simulink model "L3Pilot_ADF_v1"  (R2018b)
settings: Solver=FixedStepAuto  StartTime=0.0  StopTime=350  RelTol=1e-3  EnableMultiTasking=on
values from neighbouring files (symbols this model uses):
  a_x_MRM_critical = 5    [Var_L3Pilot_ADF_v1.m]
  a_x_MRM_normal = 2    [Var_L3Pilot_ADF_v1.m]
  Distance_forced_lane_change = 10    [Var_L3Pilot_ADF_v1.m]
  K_d_value_100 = 0.09    [Var_L3Pilot_ADF_v1.m]
  K_d_value_130 = 0.08    [Var_L3Pilot_ADF_v1.m]
  K_d_value_60 = 0.1    [Var_L3Pilot_ADF_v1.m]
  K_i_value_100 = 1    [Var_L3Pilot_ADF_v1.m]
  K_i_value_130 = 1    [Var_L3Pilot_ADF_v1.m]
  K_i_value_60 = 1    [Var_L3Pilot_ADF_v1.m]
  K_p_value_100 = 0.1    [Var_L3Pilot_ADF_v1.m]
  K_p_value_130 = 0.1    [Var_L3Pilot_ADF_v1.m]
  K_p_value_60 = 0.1    [Var_L3Pilot_ADF_v1.m]
  K_v1_value_100 = 0.1    [Var_L3Pilot_ADF_v1.m]
  K_v1_value_130 = 0.1    [Var_L3Pilot_ADF_v1.m]
  K_v1_value_60 = 0.1    [Var_L3Pilot_ADF_v1.m]
  K_v2_value_100 = 0.2    [Var_L3Pilot_ADF_v1.m]
  K_v2_value_130 = 0.2    [Var_L3Pilot_ADF_v1.m]
  K_v2_value_60 = 0.2    [Var_L3Pilot_ADF_v1.m]
  Set_velocity = 60/3.6    (= 16.6666666667)    [Var_L3Pilot_ADF_v1.m]
  t_MRM = 60    [Var_L3Pilot_ADF_v1.m]
  t_takeover = 70    [Var_L3Pilot_ADF_v1.m]
  Tabt = 0.1    [Var_L3Pilot_ADF_v1.m]
  x_LC_Forced_value = 99999    [Var_L3Pilot_ADF_v1.m]
undefined symbols (not defined in the file or in its folder): ComponentState
libraries: simulink x2
(part 1 of 2)
settings Model: Creator=QXV8396  LastModifiedBy=Q395473
settings DataIOCC: LimitDataPoints=on
settings DebuggingCC: AllowSymbolicDim=off  SFUnexpectedBacktrackingDiag=warning  SFNoUnconditionalDefaultTransitionDiag=warning  SFExecutionAtInitializationDiag=none
settings ModelReferenceCC: PropagateSignalLabelsOutOfModel=off
settings SFSimCC: SimUseLocalCustomCode=off
settings RTWCC: SystemTargetFile=fmu_cs1.tlc  MakeCommand=make_rtw FMIT_INTERMEDIATE_LIB_DIR=DEFAULT FMIT_ADDITIONAL_CFLAGS=  TemplateMakefile=fmu_cs1_default_tmf  Description=FMU Co-Simulation 1.0 Standalone  RTWUseLocalCustomCode=off
settings CodeAppCC: StateflowObjectComments=on
settings STFCustomTargetCC: ModelReferenceCompliant=off  MultiInstanceERTCode=on  CodeInterfacePackaging=Reusable function  MATLABClassNameForMDSCustomization=Simulink.SoftwareTarget.TargetSpecificTriggerConfigurationBase  GRTInterface=on  GenerateAllocFcn=on  SystemTargetFile=fmu_cs1.tlc
settings ConfigComp: CovMetricSettings=dw  CovHtmlReporting=on  CovSaveCumulativeToWorkspaceVar=on  CovSaveSingleToWorkspaceVar=on  CovExternalEMLEnable=off

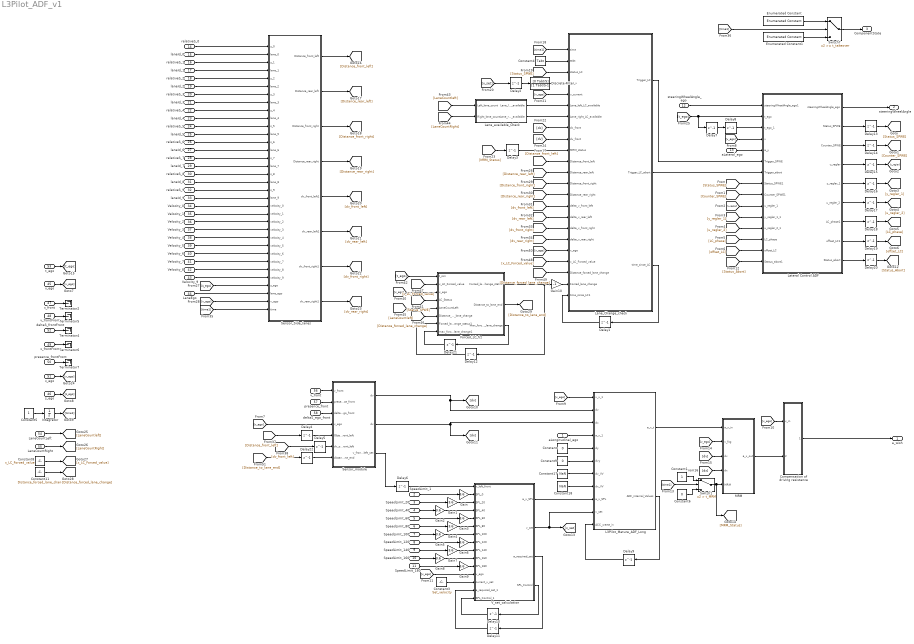
== system L3Pilot_ADF_v1 ==
  aLongitudinal_ego : Inport
  SpeedLimit_1 : Inport  Port=2  OutDataTypeStr=double
  SpeedLimit_20 : Inport  Port=3  OutDataTypeStr=double
  SpeedLimit_40 : Inport  Port=4  OutDataTypeStr=double
  SpeedLimit_60 : Inport  Port=5  OutDataTypeStr=double
  SpeedLimit_80 : Inport  Port=6  OutDataTypeStr=double
  SpeedLimit_100 : Inport  Port=7  OutDataTypeStr=double
  SpeedLimit_120 : Inport  Port=8  OutDataTypeStr=double
  SpeedLimit_140 : Inport  Port=9  OutDataTypeStr=double
  SpeedLimit_160 : Inport  Port=10  OutDataTypeStr=double
  SpeedLimit_180 : Inport  Port=11  OutDataTypeStr=double
  steeringWheelAngle_ego : Inport  Port=12
  aLateral_ego : Inport  Port=13
  relativeS_0 : Inport  Port=14  OutDataTypeStr=double
  laneId_0 : Inport  Port=15  OutDataTypeStr=int8
  relativeS_1 : Inport  Port=16  OutDataTypeStr=double
  laneId_1 : Inport  Port=17  OutDataTypeStr=int8
  relativeS_2 : Inport  Port=18  OutDataTypeStr=double
  laneId_2 : Inport  Port=19  OutDataTypeStr=int8
  relativeS_3 : Inport  Port=20  OutDataTypeStr=double
  laneId_3 : Inport  Port=21  OutDataTypeStr=int8
  relativeS_4 : Inport  Port=22  OutDataTypeStr=double
  laneId_4 : Inport  Port=23  OutDataTypeStr=int8
  relativeS_5 : Inport  Port=24  OutDataTypeStr=double
  laneId_5 : Inport  Port=25  OutDataTypeStr=int8
  relativeS_6 : Inport  Port=26  OutDataTypeStr=double
  laneId_6 : Inport  Port=27  OutDataTypeStr=int8
  relativeS_7 : Inport  Port=28  OutDataTypeStr=double
  laneId_7 : Inport  Port=29  OutDataTypeStr=int8
  relativeS_8 : Inport  Port=30  OutDataTypeStr=double
  laneId_8 : Inport  Port=31  OutDataTypeStr=int8
  relativeS_9 : Inport  Port=32  OutDataTypeStr=double
  laneId_9 : Inport  Port=33  OutDataTypeStr=int8
  Velocity_0 : Inport  Port=34  OutDataTypeStr=double
  Velocity_1 : Inport  Port=35  OutDataTypeStr=double
  Velocity_2 : Inport  Port=36  OutDataTypeStr=double
  Velocity_3 : Inport  Port=37  OutDataTypeStr=double
  Velocity_4 : Inport  Port=38  OutDataTypeStr=double
  Velocity_5 : Inport  Port=39  OutDataTypeStr=double
  Velocity_6 : Inport  Port=40  OutDataTypeStr=double
  Velocity_7 : Inport  Port=41  OutDataTypeStr=double
  Velocity_8 : Inport  Port=42  OutDataTypeStr=double
  Velocity_9 : Inport  Port=43  OutDataTypeStr=double
  LaneEgo : Inport  Port=44  OutDataTypeStr=int8
  v_ego : Inport  Port=45  OutDataTypeStr=double
  s_ego : Inport  Port=46
  x_front : Inport  Port=47  OutDataTypeStr=double
  v_frontFront : Inport  Port=48  OutDataTypeStr=double
  x_frontFront : Inport  Port=49  OutDataTypeStr=double
  presence_frontFront : Inport  Port=50  OutDataTypeStr=boolean
  x_ego : Inport  Port=51
  deltaS_frontFront : Inport  Port=52  OutDataTypeStr=double
  t_ego : Inport  Port=53
  LaneCountLeft : Inport  Port=54  OutDataTypeStr=int8
  LaneCountRight : Inport  Port=55  OutDataTypeStr=int8
  v_front : Inport  Port=56  OutDataTypeStr=double
  presence_front : Inport  Port=57  OutDataTypeStr=boolean
  deltaS_ego_front : Inport  Port=58
  Compensation of driving resistance : Subsystem
  Constant : Constant  Value=0  SampleTime=Tabt
  Constant1 : Constant  SampleTime=Tabt
  Constant11 : Constant  Value=Distance_forced_lane_change  SampleTime=Tabt
  Constant17 : Constant  Value=NaN  SampleTime=Tabt
  Constant18 : Constant  Value=NaN  SampleTime=Tabt
  Constant3 : Constant  Value=Set_velocity  SampleTime=Tabt
  Constant4 : Constant  Value=Tabt
  Constant5 : Constant  SampleTime=Tabt
  Constant6 : Constant  Value=0  SampleTime=Tabt
  Constant8 : Constant  Value=x_LC_Forced_value  SampleTime=Tabt
  Constant9 : Constant  Value=0  SampleTime=Tabt
  Delay{1..8,12..22} (19 alike) : Delay  DelayLength=1  InitialCondition=0  SampleTime=0.1
  Delay10 : Delay  DelayLength=1  InitialCondition=0  SampleTime=Tabt
  Delay11 : Delay  DelayLength=1  InitialCondition=0  SampleTime=Tabt
  Delay9 : Delay  DelayLength=1  InitialCondition=0  SampleTime=Tabt
  Discrete Filter : DiscreteFilter  Numerator=[0 Tabt/5]  Denominator=[1 Tabt/5-1]
  Enumerated Constant : simulink/Sources/Enumerated Constant  OutDataTypeStr=Enum: ComponentState  Value=ComponentState.Disabled  SampleTime=inf
      settings: SourceProductName=Simulink
  Enumerated Constant1 : simulink/Sources/Enumerated Constant  OutDataTypeStr=Enum: ComponentState  Value=ComponentState.Acting  SampleTime=inf
      settings: SourceProductName=Simulink
  Forced_LC_fct : MATLAB Function  TreatAsAtomicUnit=on
  Gain{,1..9} (10 alike) : Gain  Gain=3.6
  Gain10 : Gain  Gain=-1
  Integrator : Integrator
  L3Pilot_Mature_ADF_Long : Subsystem
  Lane_Change_check : MATLAB Function  TreatAsAtomicUnit=on
  Lane_available_Check : Subsystem
  Lateral Control ADF : MATLAB Function  TreatAsAtomicUnit=on
  MRM : Subsystem
  Sensor_Side_lanes : Subsystem
  Sensor_module : Subsystem
  Switch1 : Switch  Criteria=u2 > Threshold  Threshold=t_MRM
  Switch7 : Switch  Threshold=t_takeover
  Terminator{2,4..7} (5 alike) : Terminator
  V_set_calculation : MATLAB Function  TreatAsAtomicUnit=on
  a_wish : Outport
  steeringWheelAngle : Outport  Port=2
  ComponentState : Outport  Port=3  OutDataTypeStr=Enum: ComponentState
  wires:
  Constant17/1 -> L3Pilot_Mature_ADF_Long/7(dv_VV)
  Constant18/1 -> L3Pilot_Mature_ADF_Long/8(dx_VV)
  Constant9/1 -> L3Pilot_Mature_ADF_Long/6(dvy)
  L3Pilot_Mature_ADF_Long/1(a_x_t) -> MRM/1(a_x_in)
  Constant/1 -> L3Pilot_Mature_ADF_Long/5(dy)
  Delay9/1 -> L3Pilot_Mature_ADF_Long/11(ACC_werte_in)
  aLongitudinal_ego/1 -> L3Pilot_Mature_ADF_Long/4("a_x_1 ")
  L3Pilot_Mature_ADF_Long/2(ADF_internal_Values) -> Delay9/1
  [v_ego] -> L3Pilot_Mature_ADF_Long/1(v_x_1)
  [v_ego] -> Compensation of driving resistance/1(v_in)
  Sensor_module/1(dv) -> L3Pilot_Mature_ADF_Long/2(dv), [dv]
  Sensor_module/2(dx) -> L3Pilot_Mature_ADF_Long/3(dx), [dx]
  V_set_calculation/2(v_set) -> L3Pilot_Mature_ADF_Long/10(v_set), [v_set]
  Delay10/1 -> V_set_calculation/15(SPL_Control_1)
  Constant1/1 -> Switch1/1
  [time1] -> Switch1/2
  Constant6/1 -> Switch1/3
  Switch1/1 -> [MRM_Status], MRM/5(MRM)
  MRM/1(a_x_out) -> Compensation of driving resistance/2(a_x_in)
  [v_ego] -> MRM/2(v_fzg)
  [dx] -> MRM/4(dx)
  [dv] -> MRM/3(dv)
  V_set_calculation/4(SPL_Control) -> Delay10/1
  V_set_calculation/3(a_required_set) -> Delay11/1
  Delay11/1 -> V_set_calculation/14(a_required_set_1)
  [v_ego] -> V_set_calculation/12(v_ego)
  SpeedLimit_1/1 -> Gain/1
  SpeedLimit_20/1 -> Gain1/1
  SpeedLimit_40/1 -> Gain2/1
  SpeedLimit_60/1 -> Gain3/1
  SpeedLimit_80/1 -> Gain4/1
  SpeedLimit_100/1 -> Gain5/1
  SpeedLimit_120/1 -> Gain6/1
  SpeedLimit_160/1 -> Gain8/1
  SpeedLimit_180/1 -> Gain9/1
  SpeedLimit_140/1 -> Gain7/1
  Constant3/1 -> V_set_calculation/13(current_v_set)
  V_set_calculation/1(a_x_SPL) -> L3Pilot_Mature_ADF_Long/9(a_x_SPL)
  Gain/1 -> V_set_calculation/2(SPL_0)
  Gain1/1 -> V_set_calculation/3(SPL_20)
  Gain2/1 -> V_set_calculation/4(SPL_40)
  Gain3/1 -> V_set_calculation/5(SPL_60)
  Gain4/1 -> V_set_calculation/6(SPL_80)
  Gain5/1 -> V_set_calculation/7(SPL_100)
  Gain6/1 -> V_set_calculation/8(SPL_120)
  Gain7/1 -> V_set_calculation/9(SPL_140)
  Gain8/1 -> V_set_calculation/10(SPL_160)
  Gain9/1 -> V_set_calculation/11(SPL_180)
  Sensor_module/3(v_front_left_set) -> Delay6/1
  Delay6/1 -> V_set_calculation/1(v_left_front)
  Compensation of driving resistance/1(a_x_out) -> a_wish/1
  [t_ego] -> Forced_LC_fct/1(t_sim)
  [LaneCountleft] -> Lane_available_Check/1(Left_lane_count)
  Gain10/1 -> Lane_Change_check/22(Forced_lane_change)
  relativeS_1/1 -> Sensor_Side_lanes/3(s_1)
  Delay21/1 -> Forced_LC_fct/8(max_force_lane_change1)
  Velocity_2/1 -> Sensor_Side_lanes/23(velocity_2)
  laneId_9/1 -> Sensor_Side_lanes/20(lane_9)
  Forced_LC_fct/3(max_force_lane_change) -> Delay21/1
  relativeS_4/1 -> Sensor_Side_lanes/9(s_4)
  [dv] -> Lane_Change_check/9(dv_front)
  [Status_SPWE] -> Forced_LC_fct/4(LC_Status)
  Forced_LC_fct/1(Forced_lane_change_status) -> Delay12/1, Gain10/1
  Lateral Control ADF/4(u_regler) -> Delay15/1
  Delay12/1 -> Forced_LC_fct/7(Forced_lane_change_status1)
  [time1] -> Switch7/2
  Constant4/1 -> Lane_Change_check/2(tabt)
  [Distance_rear_left] -> Lane_Change_check/12(Distance_rear_left)
  Velocity_4/1 -> Sensor_Side_lanes/25(velocity_4)
  [Distance_rear_right] -> Lane_Change_check/14(Distance_rear_right)
  [dv_front_right] -> Lane_Change_check/17(delta_v_front_right)
  Sensor_Side_lanes/4(Distance_rear_right) -> [Distance_rear_right]
  Sensor_Side_lanes/2(Distance_rear_left) -> [Distance_rear_left]
  [time1] -> Lane_Change_check/1(time)
  Switch7/1 -> ComponentState/1
  [Status_Abort] -> Lateral Control ADF/15(Status_abort1)
  Lateral Control ADF/3(Counter_SPWE) -> Delay14/1
  Sensor_Side_lanes/6(dv_rear_left1) -> [dv_rear_left]
  Velocity_8/1 -> Sensor_Side_lanes/29(velocity_8)
  Velocity_9/1 -> Sensor_Side_lanes/30(velocity_9)
  [Distance_front_left] -> Lane_Change_check/11(Distance_front_left)
  relativeS_8/1 -> Sensor_Side_lanes/17(s_8)
  Sensor_Side_lanes/5(dv_front_left1) -> [dv_front_left]
  [Distance_front_right] -> Lane_Change_check/13(Distance_front_right)
  [v_set] -> Delay2/1
  Sensor_Side_lanes/3(Distance_front_right) -> [Distance_front_right]
  relativeS_2/1 -> Sensor_Side_lanes/5(s_2)
  relativeS_9/1 -> Sensor_Side_lanes/19(s_9)
  Velocity_1/1 -> Sensor_Side_lanes/22(velocity_1)
  Delay19/1 -> [offset_LC]
  relativeS_7/1 -> Sensor_Side_lanes/15(s_7)
  relativeS_6/1 -> Sensor_Side_lanes/13(s_6)
  relativeS_0/1 -> Sensor_Side_lanes/1(s_0)
  laneId_7/1 -> Sensor_Side_lanes/16(lane_7)
  relativeS_5/1 -> Sensor_Side_lanes/11(s_5)
  laneId_2/1 -> Sensor_Side_lanes/6(lane_2)
  laneId_3/1 -> Sensor_Side_lanes/8(lane_3)
  laneId_1/1 -> Sensor_Side_lanes/4(lane_1)
  Delay1/1 -> Lane_Change_check/23(time_since_LC1)
  Lateral Control ADF/8(offset_LC1) -> Delay19/1
  Delay3/1 -> Lane_Change_check/10(MRM_status)
  Delay14/1 -> [Counter_SPWE]
  Delay7/1 -> Delay8/1
  Delay15/1 -> [u_regler]
  Lateral Control ADF/7(LC_phase1) -> Delay18/1
  Delay20/1 -> [Status_Abort]
  Delay2/1 -> Discrete Filter/1
  [Status_SPWE] -> Lane_Change_check/3(status_LC)
  Delay16/1 -> [y_regler_1]
  [MRM_Status] -> Delay3/1
  Velocity_3/1 -> Sensor_Side_lanes/24(velocity_3)
  Lateral Control ADF/2(Status_SPWE) -> Delay13/1
  Velocity_6/1 -> Sensor_Side_lanes/27(velocity_6)
  Delay13/1 -> [Status_SPWE]
  aLateral_ego/1 -> Lateral Control ADF/5(a_y)
  [v_ego] -> Sensor_Side_lanes/33(v_ego)
  Lane_Change_check/1(Trigger_LC) -> Lateral Control ADF/6(Trigger_SPWE)
  Lateral Control ADF/6(u_regler_2) -> Delay17/1
  [u_regler_2] -> Lateral Control ADF/12(u_regler_2_1)
  LaneEgo/1 -> Sensor_Side_lanes/32(lane_ego)
  [v_ego] -> Lane_Change_check/5(v_current)
  Lateral Control ADF/5(y_regler_1) -> Delay16/1
  Velocity_7/1 -> Sensor_Side_lanes/28(velocity_7)
  [x_ego] -> Forced_LC_fct/3(x_ego)
  [y_regler_1] -> Lateral Control ADF/11(y_regler_1_1)
  [x_LC_Forced_value] -> Lane_Change_check/20(x_LC_Forced_value)
  Delay8/1 -> Lateral Control ADF/3(t_ego_1)
  [v_ego] -> Lateral Control ADF/4(v)
  Delay18/1 -> [LC_phase]
  [dv_rear_right] -> Lane_Change_check/18(delta_v_rear_right)
  Velocity_5/1 -> Sensor_Side_lanes/26(velocity_5)
  [Status_SPWE] -> Lateral Control ADF/8(Status_SPWE1)
  Lane_available_Check/1(Lane_left_LC_available) -> Lane_Change_check/6(Lane_left_LC_available)
  relativeS_3/1 -> Sensor_Side_lanes/7(s_3)
  Sensor_Side_lanes/1(Distance_front_left) -> [Distance_front_left]
  laneId_6/1 -> Sensor_Side_lanes/14(lane_6)
  [x_LC_Forced_value] -> Forced_LC_fct/2(x_LC_Forced_value)
  [offset_LC] -> Lateral Control ADF/14(offset_LC)
  Delay17/1 -> [u_regler_2]
  [t_ego] -> Delay7/1, Lateral Control ADF/2(t_ego)
  Lane_available_Check/2(Lane_right_LC_available) -> Lane_Change_check/7(Lane_right_LC_available)
  [LaneCountRight] -> Lane_available_Check/2(Right_lane_count)
  Lane_Change_check/3(time_since_LC) -> Delay1/1
  [x_ego] -> Lane_Change_check/19(x_ego)
  Lateral Control ADF/9(Status_abort) -> Delay20/1
  [dv_front_left] -> Lane_Change_check/15(delta_v_front_left)
  Sensor_Side_lanes/8(dv_rear_right1) -> [dv_rear_right]
  Lateral Control ADF/1(steeringWheelAngle_ego) -> steeringWheelAngle/1
  Lane_Change_check/2(Trigger_LC_abort) -> Lateral Control ADF/7(Trigger_abort)
  laneId_8/1 -> Sensor_Side_lanes/18(lane_8)
  [time1] -> Sensor_Side_lanes/34(time)
  [LC_phase] -> Lateral Control ADF/13(LC_phase)
  Discrete Filter/1 -> Lane_Change_check/4(set_v)
  [u_regler] -> Lateral Control ADF/10(u_regler_1)
  [dx] -> Lane_Change_check/8(dx_front)
  [dv_rear_left] -> Lane_Change_check/16(delta_v_rear_left)
  [Distance_forced_lane_change] -> Forced_LC_fct/6(Distance_forced_lane_change)
  steeringWheelAngle_ego/1 -> Lateral Control ADF/1(steeringWheelAngle_ego1)
  [s_ego] -> Sensor_Side_lanes/31("s_ego ")
  Sensor_Side_lanes/7(dv_front_right1) -> [dv_front_right]
  laneId_4/1 -> Sensor_Side_lanes/10(lane_4)
  Enumerated Constant1/1 -> Switch7/3
  Enumerated Constant/1 -> Switch7/1
  Forced_LC_fct/2(Distance_to_lane_end) -> [Distance_to_lane_end]
  laneId_5/1 -> Sensor_Side_lanes/12(lane_5)
  [Counter_SPWE] -> Lateral Control ADF/9(Counter_SPWE1)
  [LaneCountleft] -> Forced_LC_fct/5(LaneCountLeft)
  [Distance_forced_lane_change] -> Lane_Change_check/21(Distance_forced_lane_change)
  laneId_0/1 -> Sensor_Side_lanes/2("lane_0 ")
  Velocity_0/1 -> Sensor_Side_lanes/21(velocity_0)
  x_front/1 -> Terminator2/1
  t_ego/1 -> [t_ego]
  x_frontFront/1 -> Terminator6/1
  x_ego/1 -> [x_ego]
  Integrator/1 -> [time1]
  s_ego/1 -> [s_ego]
  Constant5/1 -> Integrator/1
  deltaS_frontFront/1 -> Terminator4/1
  LaneCountLeft/1 -> [LaneCountleft]
  LaneCountRight/1 -> [LaneCountRight]
  v_frontFront/1 -> Terminator5/1
  Constant8/1 -> [x_LC_Forced_value]
  v_ego/1 -> [v_ego]
  Constant11/1 -> [Distance_forced_lane_change]
  presence_frontFront/1 -> Terminator7/1
  Delay4/1 -> Sensor_module/5("Object_front_left ")
  Delay5/1 -> Sensor_module/6(dv_object_front_left)
  v_front/1 -> Sensor_module/1(v_front)
  [v_ego] -> Sensor_module/4(v_ego)
  presence_front/1 -> Sensor_module/2(presence_front)
  [Distance_to_lane_end] -> Delay22/1
  [dv_front_left] -> Delay5/1
  Delay22/1 -> Sensor_module/7(distance_lane_end)
  deltaS_ego_front/1 -> Sensor_module/3(deltaS_ego_front)
  [Distance_front_left] -> Delay4/1

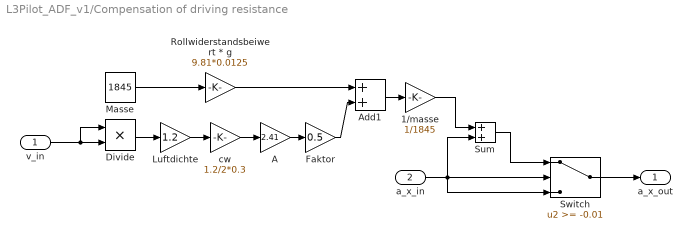
== system L3Pilot_ADF_v1/Compensation of driving resistance ==
  v_in : Inport
  a_x_in : Inport  Port=2
  1/masse : Gain  Gain=1/1845
  A : Gain  Gain=2.41  OutDataTypeStr=double
  Add1 : Sum
  Divide : Product  Inputs=**
  Faktor : Gain  Gain=0.5  OutDataTypeStr=double
  Luftdichte : Gain  Gain=1.2  OutDataTypeStr=double
  Masse : Constant  Value=1845
  Rollwiderstandsbeiwert * g : Gain  Gain=9.81*0.0125
  Sum : Sum
  Switch : Switch  Threshold=-0.01
  cw : Gain  Gain=1.2/2*0.3  OutDataTypeStr=double
  a_x_out : Outport
  wires:
  Divide/1 -> Luftdichte/1
  Add1/1 -> 1/masse/1
  a_x_in/1 -> Sum/2, Switch/3, Switch/2
  Switch/1 -> a_x_out/1
  Masse/1 -> Rollwiderstandsbeiwert * g/1
  v_in/1 -> Divide/1, Divide/2
  1/masse/1 -> Sum/1
  Sum/1 -> Switch/1
  Rollwiderstandsbeiwert * g/1 -> Add1/1
  cw/1 -> A/1
  Luftdichte/1 -> cw/1
  A/1 -> Faktor/1
  Faktor/1 -> Add1/2

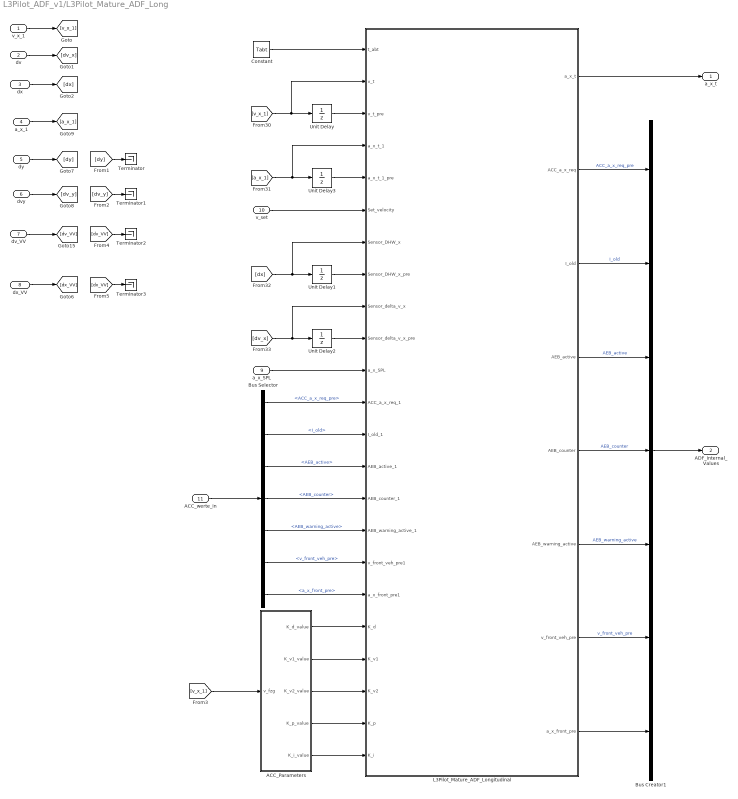
== system L3Pilot_ADF_v1/L3Pilot_Mature_ADF_Long ==
  v_x_1 : Inport
  dv : Inport  Port=2
  dx : Inport  Port=3
  "a_x_1 " : Inport  Port=4
  dy : Inport  Port=5
  dvy : Inport  Port=6
  dv_VV : Inport  Port=7
  dx_VV : Inport  Port=8
  a_x_SPL : Inport  Port=9
  v_set : Inport  Port=10
  ACC_werte_in : Inport  Port=11
  ACC_Parameters : Subsystem
  Bus Creator1 : BusCreator  Inputs=7
  Bus Selector : BusSelector  OutputSignals=ACC_a_x_req_pre,I_old,AEB_active,AEB_counter,AEB_warning_active,v_front_veh_pre,a_x_front_pre
  Constant : Constant  Value=Tabt
  L3Pilot_Mature_ADF_Longitudinal : MATLAB Function  TreatAsAtomicUnit=on
  Terminator{,1..3} (4 alike) : Terminator
  Unit Delay{,1..3} (4 alike) : UnitDelay  SampleTime=-1
  a_x_t : Outport
  ADF_internal_Values : Outport  Port=2
  wires:
  v_x_1/1 -> [v_x_1]
  dv/1 -> [dv_x]
  dx/1 -> [dx]
  dy/1 -> [dy]
  dvy/1 -> [dv_y]
  "a_x_1 "/1 -> [a_x_1]
  Bus Creator1/1 -> ADF_internal_Values/1
  ACC_werte_in/1 -> Bus Selector/1
  Constant/1 -> L3Pilot_Mature_ADF_Longitudinal/1(t_abt)
  [v_x_1] -> L3Pilot_Mature_ADF_Longitudinal/2(v_t), Unit Delay/1
  Unit Delay/1 -> L3Pilot_Mature_ADF_Longitudinal/3(v_t_pre)
  [a_x_1] -> L3Pilot_Mature_ADF_Longitudinal/4(a_x_t_1), Unit Delay3/1
  v_set/1 -> L3Pilot_Mature_ADF_Longitudinal/6(Set_velocity)
  L3Pilot_Mature_ADF_Longitudinal/1(a_x_t) -> a_x_t/1
  [dx] -> L3Pilot_Mature_ADF_Longitudinal/7(Sensor_DHW_x), Unit Delay1/1
  [dv_x] -> L3Pilot_Mature_ADF_Longitudinal/9(Sensor_delta_v_x), Unit Delay2/1
  Unit Delay1/1 -> L3Pilot_Mature_ADF_Longitudinal/8(Sensor_DHW_x_pre)
  Unit Delay2/1 -> L3Pilot_Mature_ADF_Longitudinal/10(Sensor_delta_v_x_pre)
  dx_VV/1 -> [dx_VV]
  dv_VV/1 -> [dv_VV]
  L3Pilot_Mature_ADF_Longitudinal/2(ACC_a_x_req) -> Bus Creator1/1  "ACC_a_x_req_pre"
  Bus Selector/2 -> L3Pilot_Mature_ADF_Longitudinal/13(I_old_1)  "<I_old>"
  [dy] -> Terminator/1
  [dv_y] -> Terminator1/1
  L3Pilot_Mature_ADF_Longitudinal/3(I_old) -> Bus Creator1/2  "I_old"
  Bus Selector/1 -> L3Pilot_Mature_ADF_Longitudinal/12(ACC_a_x_req_1)  "<ACC_a_x_req_pre>"
  ACC_Parameters/1(K_d_value) -> L3Pilot_Mature_ADF_Longitudinal/19(K_d)
  ACC_Parameters/2(K_v1_value) -> L3Pilot_Mature_ADF_Longitudinal/20(K_v1)
  ACC_Parameters/3(K_v2_value) -> L3Pilot_Mature_ADF_Longitudinal/21(K_v2)
  ACC_Parameters/4(K_p_value) -> L3Pilot_Mature_ADF_Longitudinal/22(K_p)
  ACC_Parameters/5(K_i_value) -> L3Pilot_Mature_ADF_Longitudinal/23(K_i)
  L3Pilot_Mature_ADF_Longitudinal/4(AEB_active) -> Bus Creator1/3  "AEB_active"
  L3Pilot_Mature_ADF_Longitudinal/5(AEB_counter) -> Bus Creator1/4  "AEB_counter"
  Bus Selector/3 -> L3Pilot_Mature_ADF_Longitudinal/14(AEB_active_1)  "<AEB_active>"
  Bus Selector/4 -> L3Pilot_Mature_ADF_Longitudinal/15(AEB_counter_1)  "<AEB_counter>"
  Unit Delay3/1 -> L3Pilot_Mature_ADF_Longitudinal/5(a_x_t_1_pre)
  L3Pilot_Mature_ADF_Longitudinal/6(AEB_warning_active) -> Bus Creator1/5  "AEB_warning_active"
  Bus Selector/5 -> L3Pilot_Mature_ADF_Longitudinal/16(AEB_warning_active_1)  "<AEB_warning_active>"
  [v_x_1] -> ACC_Parameters/1(v_fzg)
  [dv_VV] -> Terminator2/1
  [dx_VV] -> Terminator3/1
  L3Pilot_Mature_ADF_Longitudinal/7(v_front_veh_pre) -> Bus Creator1/6  "v_front_veh_pre"
  Bus Selector/6 -> L3Pilot_Mature_ADF_Longitudinal/17(v_front_veh_pre1)  "<v_front_veh_pre>"
  L3Pilot_Mature_ADF_Longitudinal/8(a_x_front_pre) -> Bus Creator1/7
  Bus Selector/7 -> L3Pilot_Mature_ADF_Longitudinal/18(a_x_front_pre1)  "<a_x_front_pre>"
  a_x_SPL/1 -> L3Pilot_Mature_ADF_Longitudinal/11(a_x_SPL)

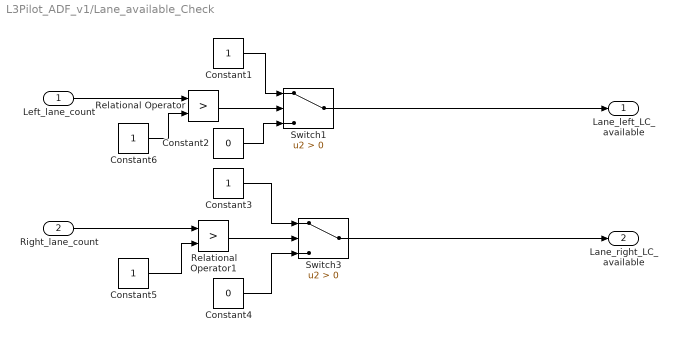
== system L3Pilot_ADF_v1/Lane_available_Check ==
  Left_lane_count : Inport
  Right_lane_count : Inport  Port=2
  Constant{1,3,5..6} (4 alike) : Constant  SampleTime=Tabt
  Constant2 : Constant  Value=0  SampleTime=Tabt
  Constant4 : Constant  Value=0  SampleTime=Tabt
  Relational Operator : RelationalOperator  Operator=>  OutDataTypeStr=boolean  RndMeth=Simplest
  Relational Operator1 : RelationalOperator  Operator=>  OutDataTypeStr=boolean  RndMeth=Simplest
  Switch1 : Switch  Criteria=u2 > Threshold
  Switch3 : Switch  Criteria=u2 > Threshold
  Lane_left_LC_available : Outport
  Lane_right_LC_available : Outport  Port=2
  wires:
  Constant2/1 -> Switch1/3
  Constant1/1 -> Switch1/1
  Constant3/1 -> Switch3/1
  Constant4/1 -> Switch3/3
  Constant6/1 -> Relational Operator/2
  Relational Operator/1 -> Switch1/2
  Relational Operator1/1 -> Switch3/2
  Constant5/1 -> Relational Operator1/2
  Right_lane_count/1 -> Relational Operator1/1
  Left_lane_count/1 -> Relational Operator/1
  Switch1/1 -> Lane_left_LC_available/1
  Switch3/1 -> Lane_right_LC_available/1

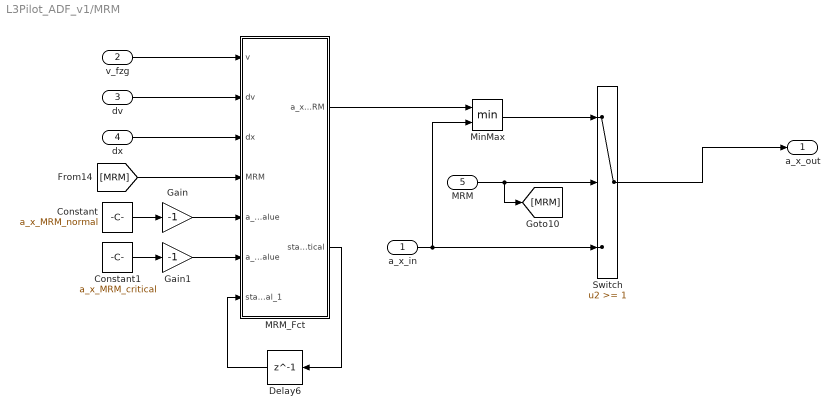
== system L3Pilot_ADF_v1/MRM ==
  a_x_in : Inport
  v_fzg : Inport  Port=2
  dv : Inport  Port=3
  dx : Inport  Port=4
  MRM : Inport  Port=5
  Constant : Constant  Value=a_x_MRM_normal  SampleTime=Tabt
  Constant1 : Constant  Value=a_x_MRM_critical  SampleTime=Tabt
  Delay6 : Delay  DelayLength=1  InitialCondition=0  SampleTime=0.1
  Gain : Gain  Gain=-1
  Gain1 : Gain  Gain=-1
  MRM_Fct : MATLAB Function  TreatAsAtomicUnit=on
  MinMax : MinMax  Inputs=2
  Switch : Switch  Threshold=1
  a_x_out : Outport
  wires:
  MRM/1 -> [MRM], Switch/2
  Switch/1 -> a_x_out/1
  a_x_in/1 -> MinMax/2, Switch/3
  MinMax/1 -> Switch/1
  MRM_Fct/1(a_x_MRM) -> MinMax/1
  v_fzg/1 -> MRM_Fct/1(v)
  dv/1 -> MRM_Fct/2(dv)
  dx/1 -> MRM_Fct/3(dx)
  [MRM] -> MRM_Fct/4(MRM)
  MRM_Fct/2(status_critical) -> Delay6/1
  Delay6/1 -> MRM_Fct/7(status_critical_1)
  Constant/1 -> Gain/1
  Constant1/1 -> Gain1/1
  Gain/1 -> MRM_Fct/5(a_x_MRM_normal_value)
  Gain1/1 -> MRM_Fct/6(a_x_MRM_critical_value)

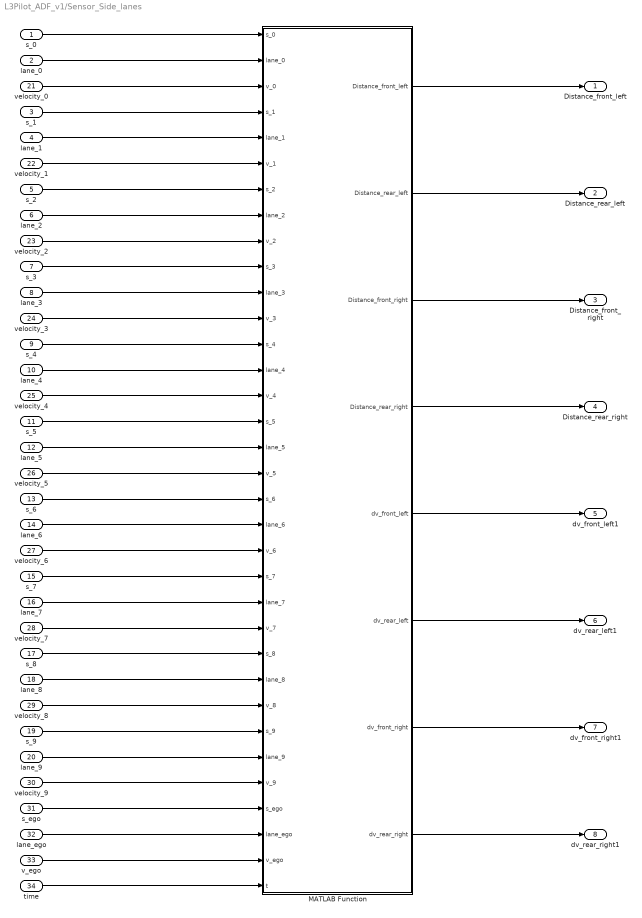
== system L3Pilot_ADF_v1/Sensor_Side_lanes ==
  s_0 : Inport
  "lane_0 " : Inport  Port=2
  s_1 : Inport  Port=3
  lane_1 : Inport  Port=4
  s_2 : Inport  Port=5
  lane_2 : Inport  Port=6
  s_3 : Inport  Port=7
  lane_3 : Inport  Port=8
  s_4 : Inport  Port=9
  lane_4 : Inport  Port=10
  s_5 : Inport  Port=11
  lane_5 : Inport  Port=12
  s_6 : Inport  Port=13
  lane_6 : Inport  Port=14
  s_7 : Inport  Port=15
  lane_7 : Inport  Port=16
  s_8 : Inport  Port=17
  lane_8 : Inport  Port=18
  s_9 : Inport  Port=19
  lane_9 : Inport  Port=20
  velocity_0 : Inport  Port=21
  velocity_1 : Inport  Port=22
  velocity_2 : Inport  Port=23
  velocity_3 : Inport  Port=24
  velocity_4 : Inport  Port=25
  velocity_5 : Inport  Port=26
  velocity_6 : Inport  Port=27
  velocity_7 : Inport  Port=28
  velocity_8 : Inport  Port=29
  velocity_9 : Inport  Port=30
  "s_ego " : Inport  Port=31
  lane_ego : Inport  Port=32
  v_ego : Inport  Port=33
  time : Inport  Port=34
  MATLAB Function : MATLAB Function  TreatAsAtomicUnit=on
  Distance_front_left : Outport
  Distance_rear_left : Outport  Port=2
  Distance_front_right : Outport  Port=3
  Distance_rear_right : Outport  Port=4
  dv_front_left1 : Outport  Port=5
  dv_rear_left1 : Outport  Port=6
  dv_front_right1 : Outport  Port=7
  dv_rear_right1 : Outport  Port=8
  wires:
  MATLAB Function/1(Distance_front_left) -> Distance_front_left/1
  MATLAB Function/2(Distance_rear_left) -> Distance_rear_left/1
  MATLAB Function/3(Distance_front_right) -> Distance_front_right/1
  MATLAB Function/4(Distance_rear_right) -> Distance_rear_right/1
  MATLAB Function/5(dv_front_left) -> dv_front_left1/1
  MATLAB Function/6(dv_rear_left) -> dv_rear_left1/1
  MATLAB Function/7(dv_front_right) -> dv_front_right1/1
  MATLAB Function/8(dv_rear_right) -> dv_rear_right1/1
  s_0/1 -> MATLAB Function/1(s_0)
  "lane_0 "/1 -> MATLAB Function/2(lane_0)
  s_1/1 -> MATLAB Function/4(s_1)
  lane_1/1 -> MATLAB Function/5(lane_1)
  s_2/1 -> MATLAB Function/7(s_2)
  lane_2/1 -> MATLAB Function/8(lane_2)
  s_3/1 -> MATLAB Function/10(s_3)
  lane_3/1 -> MATLAB Function/11(lane_3)
  s_4/1 -> MATLAB Function/13(s_4)
  lane_4/1 -> MATLAB Function/14(lane_4)
  s_5/1 -> MATLAB Function/16(s_5)
  lane_5/1 -> MATLAB Function/17(lane_5)
  s_6/1 -> MATLAB Function/19(s_6)
  lane_6/1 -> MATLAB Function/20(lane_6)
  s_7/1 -> MATLAB Function/22(s_7)
  lane_7/1 -> MATLAB Function/23(lane_7)
  s_8/1 -> MATLAB Function/25(s_8)
  lane_8/1 -> MATLAB Function/26(lane_8)
  s_9/1 -> MATLAB Function/28(s_9)
  lane_9/1 -> MATLAB Function/29(lane_9)
  "s_ego "/1 -> MATLAB Function/31(s_ego)
  lane_ego/1 -> MATLAB Function/32(lane_ego)
  velocity_0/1 -> MATLAB Function/3(v_0)
  velocity_1/1 -> MATLAB Function/6(v_1)
  velocity_2/1 -> MATLAB Function/9(v_2)
  velocity_3/1 -> MATLAB Function/12(v_3)
  velocity_4/1 -> MATLAB Function/15(v_4)
  velocity_5/1 -> MATLAB Function/18(v_5)
  velocity_6/1 -> MATLAB Function/21(v_6)
  velocity_7/1 -> MATLAB Function/24(v_7)
  velocity_8/1 -> MATLAB Function/27(v_8)
  velocity_9/1 -> MATLAB Function/30(v_9)
  v_ego/1 -> MATLAB Function/33(v_ego)
  time/1 -> MATLAB Function/34(t)

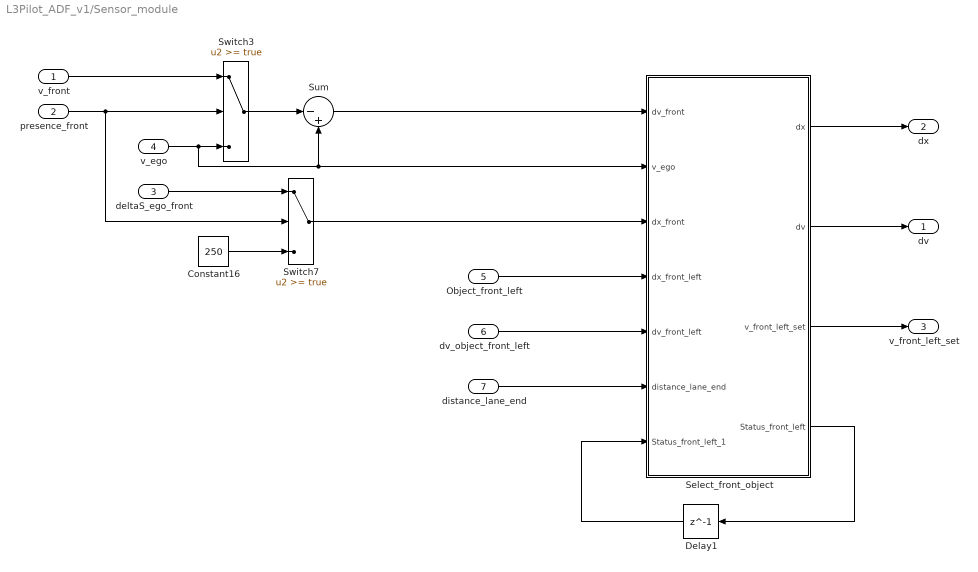
== system L3Pilot_ADF_v1/Sensor_module ==
  v_front : Inport
  presence_front : Inport  Port=2  OutDataTypeStr=boolean
  deltaS_ego_front : Inport  Port=3
  v_ego : Inport  Port=4  OutDataTypeStr=double
  "Object_front_left " : Inport  Port=5  OutDataTypeStr=double
  dv_object_front_left : Inport  Port=6  OutDataTypeStr=double
  distance_lane_end : Inport  Port=7  OutDataTypeStr=double
  Constant16 : Constant  Value=250  SampleTime=Tabt
  Delay1 : Delay  DelayLength=1  InitialCondition=0  SampleTime=0.1
  Select_front_object : MATLAB Function  TreatAsAtomicUnit=on
  Sum : Sum  Inputs=|-+
  Switch3 : Switch  Threshold=true
  Switch7 : Switch  Threshold=true
  dv : Outport
  dx : Outport  Port=2
  v_front_left_set : Outport  Port=3
  wires:
  v_front/1 -> Switch3/1
  Switch3/1 -> Sum/1
  Sum/1 -> Select_front_object/1(dv_front)
  deltaS_ego_front/1 -> Switch7/1
  presence_front/1 -> Switch7/2, Switch3/2
  Constant16/1 -> Switch7/3
  v_ego/1 -> Sum/2, Select_front_object/2(v_ego), Switch3/3
  Switch7/1 -> Select_front_object/3(dx_front)
  "Object_front_left "/1 -> Select_front_object/4(dx_front_left)
  dv_object_front_left/1 -> Select_front_object/5(dv_front_left)
  Select_front_object/1(dx) -> dx/1
  Select_front_object/2(dv) -> dv/1
  Select_front_object/3(v_front_left_set) -> v_front_left_set/1
  Select_front_object/4(Status_front_left) -> Delay1/1
  Delay1/1 -> Select_front_object/7(Status_front_left_1)
  distance_lane_end/1 -> Select_front_object/6(distance_lane_end)

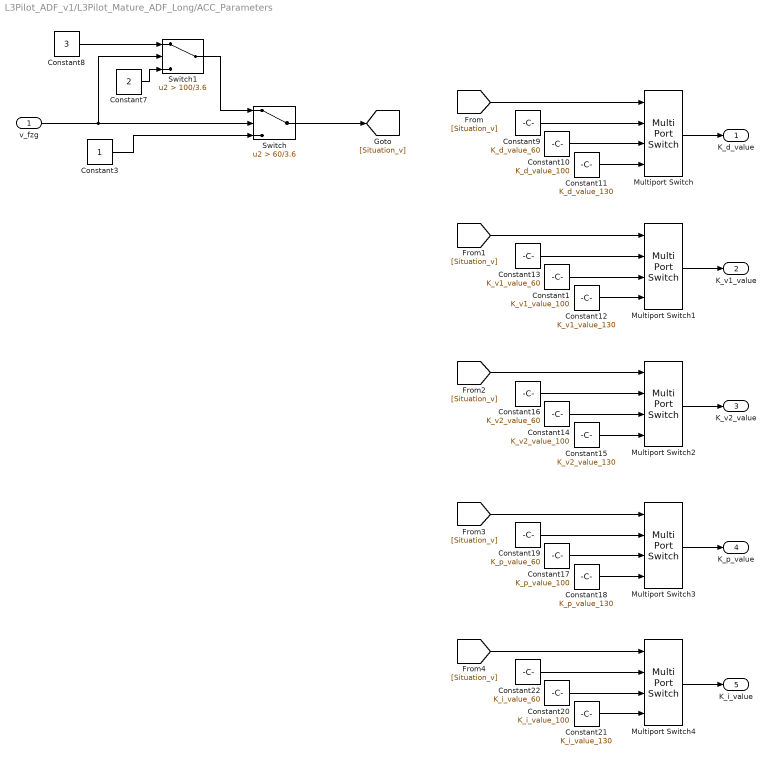
== system L3Pilot_ADF_v1/L3Pilot_Mature_ADF_Long/ACC_Parameters ==
  v_fzg : Inport
  Constant1 : Constant  Value=K_v1_value_100
  Constant10 : Constant  Value=K_d_value_100
  Constant11 : Constant  Value=K_d_value_130
  Constant12 : Constant  Value=K_v1_value_130
  Constant13 : Constant  Value=K_v1_value_60
  Constant14 : Constant  Value=K_v2_value_100
  Constant15 : Constant  Value=K_v2_value_130
  Constant16 : Constant  Value=K_v2_value_60
  Constant17 : Constant  Value=K_p_value_100
  Constant18 : Constant  Value=K_p_value_130
  Constant19 : Constant  Value=K_p_value_60
  Constant20 : Constant  Value=K_i_value_100
  Constant21 : Constant  Value=K_i_value_130
  Constant22 : Constant  Value=K_i_value_60
  Constant3 : Constant
  Constant7 : Constant  Value=2
  Constant8 : Constant  Value=3
  Constant9 : Constant  Value=K_d_value_60
  Multiport Switch{,1..4} (5 alike) : MultiPortSwitch
  Switch : Switch  Criteria=u2 > Threshold  Threshold=60/3.6
  Switch1 : Switch  Criteria=u2 > Threshold  Threshold=100/3.6
  K_d_value : Outport
  K_v1_value : Outport  Port=2
  K_v2_value : Outport  Port=3
  K_p_value : Outport  Port=4
  K_i_value : Outport  Port=5
  wires:
  v_fzg/1 -> Switch/2, Switch1/2
  Constant3/1 -> Switch/3
  Constant7/1 -> Switch1/3
  Constant8/1 -> Switch1/1
  Switch1/1 -> Switch/1
  Switch/1 -> [Situation_v]
  [Situation_v] -> Multiport Switch/1
  Constant9/1 -> Multiport Switch/2
  Constant10/1 -> Multiport Switch/3
  Constant11/1 -> Multiport Switch/4
  Multiport Switch/1 -> K_d_value/1
  [Situation_v] -> Multiport Switch1/1
  Constant13/1 -> Multiport Switch1/2
  Constant1/1 -> Multiport Switch1/3
  Constant12/1 -> Multiport Switch1/4
  Multiport Switch1/1 -> K_v1_value/1
  [Situation_v] -> Multiport Switch2/1
  Constant16/1 -> Multiport Switch2/2
  Constant14/1 -> Multiport Switch2/3
  Constant15/1 -> Multiport Switch2/4
  Multiport Switch2/1 -> K_v2_value/1
  [Situation_v] -> Multiport Switch3/1
  Constant19/1 -> Multiport Switch3/2
  Constant17/1 -> Multiport Switch3/3
  Constant18/1 -> Multiport Switch3/4
  Multiport Switch3/1 -> K_p_value/1
  [Situation_v] -> Multiport Switch4/1
  Constant22/1 -> Multiport Switch4/2
  Constant20/1 -> Multiport Switch4/3
  Constant21/1 -> Multiport Switch4/4
  Multiport Switch4/1 -> K_i_value/1

== matlab function L3Pilot_ADF_v1/V_set_calculation ==
  data: v_left_front input; SPL_0 input; a_x_SPL output; SPL_20 input; v_set output; a_required_set output; SPL_40 input; SPL_60 input; SPL_80 input; SPL_100 input; SPL_120 input; SPL_140 input; SPL_160 input; SPL_180 input; v_ego input; current_v_set input; a_required_set_1 input; SPL_Control_1 input; SPL_Control output
function [a_x_SPL,v_set,a_required_set,SPL_Control] = L3Pilot_Speed_limit...
    (v_left_front,SPL_0,SPL_20,SPL_40,SPL_60,SPL_80,SPL_100,SPL_120,SPL_140,SPL_160,SPL_180,v_ego,current_v_set,a_required_set_1,SPL_Control_1)


% a = s_ego;
% b =v_ego;
% c = current_v_set;
% 
% v_set = min([v_funct_set,speed_limit]);
% 
% a_x_SPL=NaN;

v_set = current_v_set;
a_x_SPL = NaN;
a_required_set =a_required_set_1;
SPL_Control=SPL_Control_1;

mess_SPL = 20:20:180;

[max_SPL,~] =max([SPL_20,SPL_40,SPL_60,SPL_80,SPL_100,SPL_120,SPL_140,SPL_160,SPL_180]/3.6);
[min_SPL,pos_min_SPL] =min([SPL_20,SPL_40,SPL_60,SPL_80,SPL_100,SPL_120,SPL_140,SPL_160,SPL_180]/3.6);

current_SPL = SPL_0/3.6;

if max_SPL>current_SPL
    v_set = min([current_v_set,current_SPL]); 
    a_x_SPL = NaN;
    SPL_Control =0;
else
    if min_SPL<current_SPL
        distance_new_v = mess_SPL(pos_min_SPL);
        a_required = -(v_ego.^2-min_SPL.^2)/(2*(distance_new_v-1));
        if abs(a_required)>0.5
            v_set = min([current_v_set,min_SPL]);

            if (SPL_Control_1==0) || (a_required<a_required_set_1)
                a_required_set = a_required;
            end 
                
            a_x_SPL = a_required_set;
            SPL_Control = 1;
         else
            if SPL_Control_1==0
                v_set =  nanmin([current_v_set,current_SPL,v_left_front]);
                a_x_SPL = 0;
            else
                v_set =  nanmin([current_v_set,min_SPL,v_left_front]);
                a_x_SPL = a_required_set_1;
            end
        end
    else
        v_set = nanmin([130/3.6,current_SPL,v_left_front]);  
        a_x_SPL = NaN;
        SPL_Control=0;
    end
end

if min_SPL==current_SPL
    SPL_Control = 0;
    a_required_set =0;
end

if v_ego<v_set
    SPL_Control = 0;
    a_required_set =0;
end

== matlab function L3Pilot_ADF_v1/Lateral Control ADF ==
  data: steeringWheelAngle_ego1 input; steeringWheelAngle_ego output; t_ego input; t_ego_1 input; v input; a_y input; Trigger_SPWE input; Trigger_abort input; Status_SPWE1 input; Counter_SPWE1 input; u_regler_1 input; y_regler_1_1 input; u_regler_2_1 input; LC_phase input; offset_LC input; Status_abort1 input; Status_SPWE output; Counter_SPWE output; u_regler output; y_regler_1 output; u_regler_2 output; LC_phase1 output; offset_LC1 output; Status_abort output
function [steeringWheelAngle_ego,Status_SPWE,Counter_SPWE,u_regler,y_regler_1,u_regler_2,LC_phase1,offset_LC1,Status_abort]...
    = Lateral_Control(steeringWheelAngle_ego1, t_ego, t_ego_1, v, a_y, Trigger_SPWE, Trigger_abort, Status_SPWE1,...
    Counter_SPWE1,u_regler_1,y_regler_1_1,u_regler_2_1,LC_phase,offset_LC, Status_abort1)

LC_phase1 = 0;
offset_LC1 = offset_LC;
u_regler=0;
u_regler_2 = 0;
y_regler_1 = 0;

max_steering_change = 1.5;

% KI = 0.1;
% KP = 5;
% KD  =10;

% KP = 2;
% KI = 0.0086; 
% KD  = 11.7925;

KP = 2 ;
KI = 0.1*KP * (2/3.478)*0.075;
KD  =KP*(2/0.848)*2.5;

T_SPWE_Zeit =6;

steeringWheelAngle_ego = 0;

delta_t_ego = abs(t_ego-t_ego_1)/2;
if abs(delta_t_ego)>2
    delta_t_ego = 0;
end

if abs(Trigger_SPWE)==1
    Status_SPWE = Trigger_SPWE;
else
    Status_SPWE = Status_SPWE1;
end

if Counter_SPWE1 > 20
    Status_SPWE = 0;
end

if abs(Status_SPWE) == 0 
    Counter_SPWE =0 ;
else
    Counter_SPWE = Counter_SPWE1+0.1; 
end

if v>5
    phi_current = asin(delta_t_ego/(v*0.1));
else
    phi_current = 0;
end

Status_abort = Status_abort1;
if Trigger_abort==1
    Status_abort = 1;
end

if abs(Status_SPWE) == 1 || abs(Status_abort)==1
  
    if Status_SPWE ==1
        if LC_phase ==0
            LC_phase1 =1;
            offset_LC1 = 0;
        else
            LC_phase1 = LC_phase;
            offset_LC1 = offset_LC+delta_t_ego;
        end

        d_actual_offset = t_ego;

        if t_ego < 0 && Counter_SPWE >2.5
           d_actual_offset = 3.75+t_ego;
           LC_phase1 = 2;
        end

        target_t = min([3.5,0 + 3.5/T_SPWE_Zeit*Counter_SPWE]);

        if d_actual_offset > 3.3 || Counter_SPWE>=(T_SPWE_Zeit+0.2)
            Status_SPWE=0;
        end
    
    else
         if LC_phase ==0
            LC_phase1 = 1;
            offset_LC1 = 0;
        else
            LC_phase1 = LC_phase;
            offset_LC1 = offset_LC+delta_t_ego;
        end

        d_actual_offset = t_ego;

        if t_ego > 0 && Counter_SPWE >2.5
           d_actual_offset = -3.75+t_ego;
           LC_phase1 = 2;
        end

        target_t = -1*min([3.5,0 + 3.5/T_SPWE_Zeit*Counter_SPWE]);

        if abs(d_actual_offset) > 3.3 || Counter_SPWE>=(T_SPWE_Zeit+0.2)
            Status_SPWE=0;
        end

    end
        
    if Status_abort ==1 
       if abs(d_actual_offset) < 1.5
           if Status_SPWE ==1
               target_t = 0;
           else
               target_t = 0;
           end
           if abs(d_actual_offset) < 0.25
               Status_SPWE=0;
               Status_abort = 0;
           end
           
       end
    end
    
    
    dy_vehicle = d_actual_offset;
    u_regler = (target_t-dy_vehicle);
             
    PID_Regler = (y_regler_1_1+ (KP + KI + KD)*u_regler - (KP+2*KD)*u_regler_1+(KD)*u_regler_2_1)*1;
    
%     PID_Regler =KP*u_regler*0.1;
    
    y_regler_1 = PID_Regler;
    % Begrezung des Lenkwinkels;
    delta_steering = PID_Regler-steeringWheelAngle_ego1;
    if abs(delta_steering) <= max_steering_change
        steeringWheelAngle_ego = PID_Regler;
    else
        steeringWheelAngle_ego = steeringWheelAngle_ego1+max_steering_change*sign(delta_steering);
    end
    
    u_regler_2 = u_regler_1;
    u_regler_1 = u_regler;
    
       
else
    
    sp = 2*v;
    
    dy0 = t_ego;
    
    dy_phi = tan(phi_current)*sp;
    
    phi_dot = 0;
    dy_phi_dot = 1/2 * phi_dot / v * sp^2;
    
    dy_vehicle = dy0 ;%+ dy_phi ;%+ dy_phi_dot;
    

    u_regler = (0-dy_vehicle);
             
    PID_Regler = (y_regler_1_1+ (KP + KI + KD)*u_regler - (KP+2*KD)*u_regler_1+(KD)*u_regler_2_1)*1;
    
%     PID_Regler =KP*u_regler*0.1;
    
    y_regler_1 = PID_Regler;
    
    % Begrezung des Lenkwinkels;
    delta_steering = PID_Regler-steeringWheelAngle_ego1;
    if abs(delta_steering) <= max_steering_change
        steeringWheelAngle_ego = PID_Regler;
    else
        steeringWheelAngle_ego = steeringWheelAngle_ego1+max_steering_change*sign(delta_steering);
    end
    u_regler_2 = u_regler_1;
    u_regler_1 = u_regler;
    
    offset_LC1 = 0;
    
%     steeringWheelAngle_ego = steeringWheelAngle_ego1;
end

y_regler_1_1 = steeringWheelAngle_ego;

== matlab function L3Pilot_ADF_v1/MRM/MRM_Fct ==
  data: v input; a_x_MRM output; dv input; dx input; MRM input; a_x_MRM_normal_value input; a_x_MRM_critical_value input; status_critical_1 input; status_critical output
function [a_x_MRM,status_critical] = MRM_fct(v,dv,dx,MRM,a_x_MRM_normal_value,a_x_MRM_critical_value,status_critical_1)

status_critical=0;

if (dv>0) && (dx>0)
    TTC = dx./dv;
    if TTC(1) > 10
        TTC = 10;
    end
else
    TTC = 10;
end

if MRM==0
    status_critical = 0;
else
    if TTC<3
        status_critical = 1; 
    else
        status_critical = status_critical_1; 
    end
end

if v <1
  status_critical=0;
end

if status_critical==0
    a_x_MRM = a_x_MRM_normal_value;
    
else
    a_x_MRM = a_x_MRM_critical_value;
end

== matlab function L3Pilot_ADF_v1/Sensor_module/Select_front_object ==
  data: dv_front input; dx output; v_ego input; dx_front input; dx_front_left input; dv_front_left input; distance_lane_end input; dv output; v_front_left_set output; Status_front_left_1 input; Status_front_left output
function [dx,dv,v_front_left_set,Status_front_left] = Select_front_object(dv_front, v_ego, dx_front, ...
    dx_front_left, dv_front_left,distance_lane_end,Status_front_left_1)



dx = dx_front;
dv = dv_front;

v_front_left_set = NaN;
Status_front_left = 0;

if isnan(dx_front_left) || dx_front_left<=5
    dx_front_left = 250;
    dv_front_left = 0;
end
if isnan(dv_front_left)
    dx_front_left = 0;
end

THW_threshold = 1.2;
THW_threshold_out = 1.8;
offset_front_left = 5;

THW_front_left =dx_front_left/v_ego;
THW_front_left(THW_front_left>20)=20;

% if Status_front_left_1 ==1
%     if  THW_front_left < THW_threshold
%         if (dx_front_left<dx_front) && (dv_front_left>=0.1)
%             dx = dx_front_left - offset_front_left;
%             dv = dv_front_left;
%             v_front_left_set = dv_front_left+v_ego;
%             Status_front_left = 1;
%         end
%     end
% else
%     if THW_front_left > THW_threshold_out
        Status_front_left = 0;
        dx = dx_front;
        dv = dv_front;
        v_front_left_set = NaN;     
%     else
%         dx = dx_front_left - offset_front_left;
%         dv = dv_front_left;
%         v_front_left_set = dv_front_left+v_ego;
%         Status_front_left = Status_front_left_1;
%     end
% end


% Additional Cirteria for the end of lane scenario

if distance_lane_end<=dx
    dx = distance_lane_end;
    dv = v_ego;
end

== matlab function L3Pilot_ADF_v1/Lane_Change_check ==
  data: time input; Trigger_LC output; Trigger_LC_abort output; tabt input; status_LC input; set_v input; v_current input; Lane_left_LC_available input; Lane_right_LC_available input; dx_front input; dv_front input; MRM_status input; Distance_front_left input; Distance_rear_left input; Distance_front_right input; Distance_rear_right input; delta_v_front_left input; delta_v_rear_left input; delta_v_front_right input; delta_v_rear_right input; x_ego input; x_LC_Forced_value input; Distance_forced_lane_change input; Forced_lane_change input; time_since_LC1 input; time_since_LC output
function [Trigger_LC,Trigger_LC_abort,time_since_LC] = Lane_Change_check(time,tabt,status_LC,...
    set_v,v_current, Lane_left_LC_available,Lane_right_LC_available,dx_front,dv_front,MRM_status,...
    Distance_front_left,Distance_rear_left,Distance_front_right,Distance_rear_right,...
    delta_v_front_left,delta_v_rear_left,delta_v_front_right,delta_v_rear_right,...
    x_ego,x_LC_Forced_value,Distance_forced_lane_change,Forced_lane_change,time_since_LC1)

Trigger_LC = 0;
Trigger_LC_abort = 0;
time_since_LC = time_since_LC1+tabt;
if abs(status_LC)>0
    time_since_LC = 0;
end

%%%%%%%%%%%%%%%%%%%%%%%%%%%%%%%%%%%%%%%%%%%%%%%%%%%%%%%%%%%%%%%%%%%%%%%%%%%
t_limit_LC =  15;
v_limit_trigger_LC = 10.8/3.6;
v_limit_LC = 60/3.6;

THW_front_vehicle_limit = 4;
THW_front_right_lane_free = 6;
dx_min_right_lane_free = 150;
THW_front_left_lane_free = 6;
dx_min_left_lane_free = 150;
time_out_beginning  = 13;

dx_limit_side = 10;
THW_limit_side = 1;
a_req_limt = -2;


%%%%%%%%%%%%%%%%%%%%%%%%%%%%%%%%%%%%%%%%%%%%%%%%%%%%%%%%%%%%%%%%%%%%%%%%%%%
dx_left_front = Distance_front_left;
dx_left_rear = Distance_rear_left;
dx_right_front = Distance_front_right;
dx_right_rear = Distance_rear_right;

dv_left_front = delta_v_front_left;
dv_left_rear = delta_v_rear_left;
dv_right_front = delta_v_front_right;
dv_right_rear = delta_v_rear_right;

v_rear_left = v_current-dv_left_rear;
v_rear_right = v_current-dv_right_rear;

dx_res = 5;
if (dx_left_rear-dx_res)>0
    if dv_left_rear<0 
        a_req_rear_left = 0;
    else
       a_req_rear_left = -((dv_left_rear).^2)/(2*(dx_left_rear-dx_res));
    end
else
    a_req_rear_left = -9.81;
end
if (dx_right_rear-dx_res)>0 
    if dv_right_rear<0
        a_req_rear_right = 0;
    else
        a_req_rear_right = -((dv_right_rear).^2)/(2*(dx_right_rear-dx_res));
    end
else
    a_req_rear_right = -9.81;
end
%%%%%%%%%%%%%%%%%%%%%%%%%%%%%%%%%%%%%%%%%%%%%%%%%%%%%%%%%%%%%%%%%%%%%%%%%%%

delta_v = set_v-v_current;
if v_current>2
    THW_front = dx_front / v_current;
    THW_front_left = dx_left_front / v_current;
    THW_rear_left = dx_left_rear / v_current;
    THW_front_right = dx_right_front / v_current;
    THW_rear_right = dx_right_rear / v_current;
else
    THW_front = 20;
    THW_front_left = 20;
    THW_rear_left = 20;
    THW_front_right = 20;
    THW_rear_right = 20;
end

%%%%%%%%%%%%%%%%%%%%%%%%%%%%%%%%%%%%%%%%%%%%%%%%%%%%%%%%%%%%%%%%%%%%%%%%%%%
% Criteria to start lane change

if ((THW_front_right>THW_front_right_lane_free) ||(dx_right_front > dx_min_right_lane_free))...
        && (Lane_right_LC_available==1)
     Trigger_LC = -1;
end

if ((THW_front_left>THW_front_left_lane_free) ||(dx_left_front > dx_min_left_lane_free))...
        && (Lane_left_LC_available==1)
     Trigger_LC = 1;
end

if Trigger_LC==1
    if (delta_v> v_limit_trigger_LC) && (THW_front < THW_front_vehicle_limit)
            Trigger_LC = 1;
    else
            Trigger_LC = 0;
    end
end

%%%%%%%%%%%%%%%%%%%%%%%%%%%%%%%%%%%%%%%%%%%%%%%%%%%%%%%%%%%%%%%%%%%%%%%%%%%
% Criteria to not conduct a lane change

if Trigger_LC==1
   if dx_left_front<dx_limit_side || dx_left_rear<dx_limit_side
       Trigger_LC = 0;
   end
   if THW_front_left<THW_limit_side || THW_rear_left<THW_limit_side
       Trigger_LC = 0;
   end 
   if a_req_rear_left < a_req_limt
       Trigger_LC = 0; 
   end
end

if Trigger_LC==-1
   if dx_right_front<dx_limit_side || dx_right_rear<dx_limit_side
       Trigger_LC = 0;
   end
   if THW_front_right<THW_limit_side || THW_rear_right<THW_limit_side
       Trigger_LC = 0;
   end 
   if a_req_rear_right < a_req_limt
       Trigger_LC = 0; 
   end
end

if Trigger_LC==1 && Lane_left_LC_available==0
    Trigger_LC = 0;
end
if Trigger_LC==-1 && Lane_right_LC_available==0
    Trigger_LC = 0;
end
if v_current<v_limit_LC && MRM_status==0
    Trigger_LC = 0;
end
if Trigger_LC==1 && MRM_status==1
    Trigger_LC = 0;
end


if time_since_LC<t_limit_LC
    Trigger_LC = 0;
end

if time < time_out_beginning
    Trigger_LC = 0;
end




%%%%%%%%%%%%%%%%%%%%%%%%%%%%%%%%%%%%%%%%%%%%%%%%%%%%%%%%%%%%%%%%%%%%%%%%%%%
% Addition for the end of Lane scenario

% No Lane change by the function in the area of end of lane

if  x_ego>=x_LC_Forced_value && x_ego<=(x_LC_Forced_value+Distance_forced_lane_change)
    Trigger_LC =0;
end

if abs(Forced_lane_change)>=1
    Trigger_LC = Forced_lane_change;
    
       if dx_right_front<(dx_limit_side/2) || dx_right_rear<(dx_limit_side/2)
           Trigger_LC = 0;
       end
       if THW_front_right<(THW_limit_side/4) || THW_rear_right<(THW_limit_side/4)
           Trigger_LC = 0;
       end 

else
    Trigger_LC = Trigger_LC;
end
% if time>22
%     Trigger_LC = -1;
%     if time >(15+tabt)
%         Trigger_LC = 0;
%     end
% end

%%%%%%%%%%%%%%%%%%%%%%%%%%%%%%%%%%%%%%%%%%%%%%%%%%%%%%%%%%%%%%%%%%%%%%%%%%%
% Lane Change abort
if time>999
    Trigger_LC_abort = 1;
    if time >(999+tabt)
        Trigger_LC_abort = 0;
    end
end
